simulink model "integrator_1"  (Simulink 5.0)
settings: Solver=ode45  StartTime=0.0  StopTime=10.0  RelTol=1e-3
libraries: dsparch4 x1
settings Model: Creator=svenhoffmann  LastModifiedBy=svenhoffmann  ExtModeAutoUpdateStatusClock=off

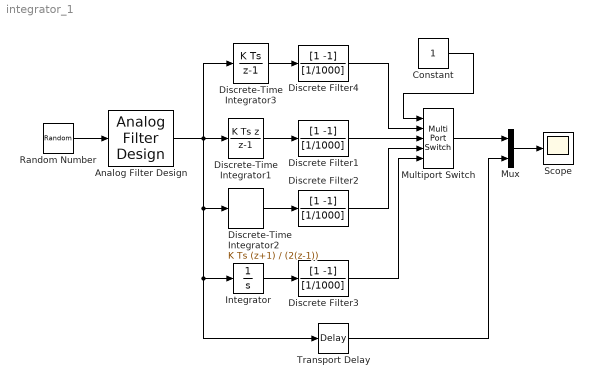
== system integrator_1 ==
  Analog Filter Design : dsparch4/Analog Filter Design  method=Butterworth  filttype=Lowpass  N=8  Wlo=2*pi*450  Whi=80  Rp=2  Rs=40
  Constant : Constant
  Discrete Filter{1..4} (4 alike) : DiscreteFilter  Numerator=[1 -1]  Denominator=[1/1000]  SampleTime=1/1000
  Discrete-Time Integrator1 : DiscreteIntegrator  IntegratorMethod=Backward Euler  SampleTime=1/1000
  Discrete-Time Integrator2 : DiscreteIntegrator  IntegratorMethod=Trapezoidal  SampleTime=1/1000
  Discrete-Time Integrator3 : DiscreteIntegrator  SampleTime=1/1000
  Integrator : Integrator
  Multiport Switch : MultiPortSwitch  SaturateOnIntegerOverflow=on
  Mux : Mux  Inputs=2
  Random Number : RandomNumber  SampleTime=0
  Scope : Scope
      settings: YMin=-1.5  YMax=1.5
  Transport Delay : TransportDelay  DelayTime=1/1000
  wires:
  Random Number/1 -> Analog Filter Design/1
  Analog Filter Design/1 -> Discrete-Time Integrator1/1, Discrete-Time Integrator2/1, Integrator/1, Transport Delay/1, Discrete-Time Integrator3/1
  Integrator/1 -> Discrete Filter3/1
  Discrete-Time Integrator2/1 -> Discrete Filter2/1
  Discrete-Time Integrator1/1 -> Discrete Filter1/1
  Mux/1 -> Scope/1
  Transport Delay/1 -> Mux/2
  Multiport Switch/1 -> Mux/1
  Discrete Filter1/1 -> Multiport Switch/3
  Discrete Filter2/1 -> Multiport Switch/4
  Discrete Filter3/1 -> Multiport Switch/5
  Constant/1 -> Multiport Switch/1
  Discrete-Time Integrator3/1 -> Discrete Filter4/1
  Discrete Filter4/1 -> Multiport Switch/2
